simulink library "sim_lib"  (R2023a)
settings: Solver=VariableStepAuto  StartTime=0.0  StopTime=10.0  RelTol=1e-3
undefined symbols (not defined in the file): DiscIntNeverNeededParam, gui, mu, simdb
libraries: $bdroot x12, dspinverses x3, matrix_library x2, simulink x1
settings Model: Creator=David  LastModifiedBy=David
settings OptimizationCC: ReuseModelBlockBuffer=off

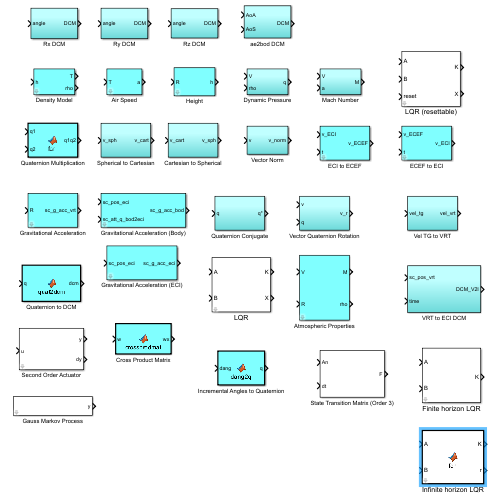
[thumbnail: Simulink's stored preview of the top-level diagram]
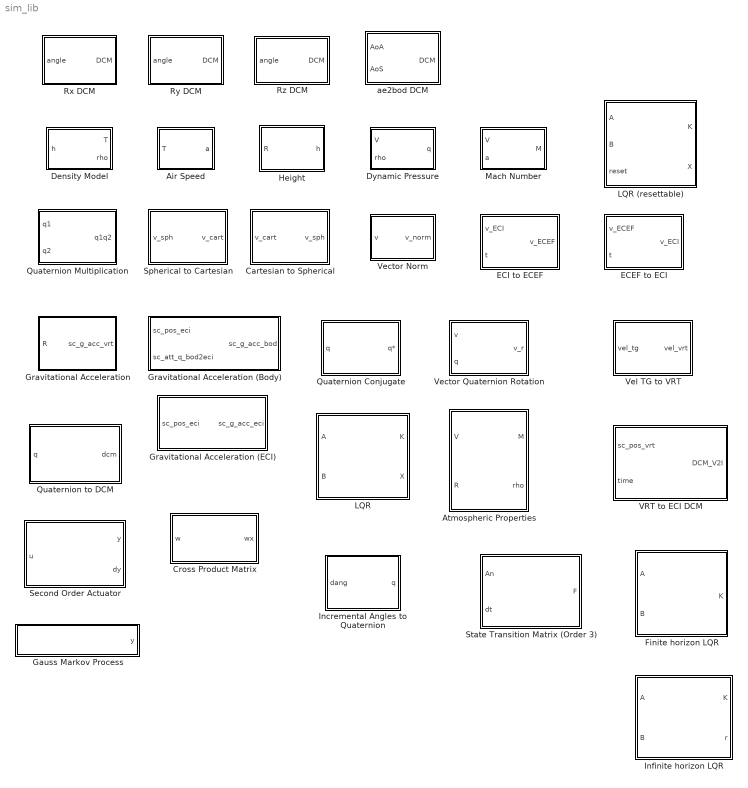
== system sim_lib ==
  Air Speed : Subsystem  mask{Rg=simdb.env.Rg, gamma=simdb.env.gamma}
      mask prompts: Rg "Gas constant"; gamma "Gas constant #2"
  Atmospheric Properties : Subsystem  mask(Atmospheric Properties){Rp=0, Rg=0, gamma=0, h_base=0, T_base=0, rho_base=0}
      mask prompts: Rp "Planet radius [m]:"; Rg "Gas constant (Rg):"; gamma "Gas constant #2 (gamma):"; h_base "Height interpolation breakpoints:"; T_base "Temperature interpolation breakpoints:"; rho_base "Density interpolation breakpoints:"
      mask help: Calculates Mach number and air density at the specified radial position and velocity.
  Cartesian to Spherical : Subsystem
  Cross Product Matrix : MATLAB Function  TreatAsAtomicUnit=on
  Density Model : Subsystem  mask{h_base=simdb.env.h_base, T_base=simdb.env.T_base, rho_base=simdb.env.rho_base}
      mask prompts: h_base "Height breakpoints"; T_base "Temperature interpolation points"; rho_base "Density interpolation points"
  Dynamic Pressure : Subsystem
  ECEF to ECI : Subsystem  mask{omega_cb=0}
      mask prompts: omega_cb "Central body rotation [rad/s]:"
  ECI to ECEF : Subsystem  mask{omega_cb=0}
      mask prompts: omega_cb "Central body rotation [rad/s]:"
  Finite horizon LQR : Subsystem  mask(Linear Quadratic Regulator){Q=gui.Q, R=gui.R, P0=eye(3), T=20, dt=0.05}
      mask prompts: Q "State cost matrix Q:"; R "Input cost matrix R:"; P0 "Initial Ricatti matrix P0:"; T "Time horizon:"; dt "Sample time:"
      mask help: Implementation of the Continuous-Time Finite-Horizon Linear Quadratic Regulator in Simulink (Compatible with Code Generator).
  Gauss Markov Process : Subsystem  mask{var=1, Tc=1, seed=0, dt=1}
      mask prompts: var "Variance:"; Tc "Autocorrelation time [s]:"; dt "Sample time [s]:"
  Gravitational Acceleration : Subsystem  mask{mu=mu}
      mask prompts: mu "Gravitational Parameter [m^3/s^2]:"
  Gravitational Acceleration (Body) : Subsystem  mask{mu=mu}
      mask prompts: mu "Gravitational Parameter [m^3/s^2]:"
  Gravitational Acceleration (ECI) : Subsystem  mask{mu=mu}
      mask prompts: mu "Gravitational Parameter [m^3/s^2]:"
  Height : Subsystem  mask{Rp=simdb.env.Rp}
      mask prompts: Rp "Planet radius"
  Incremental Angles to Quaternion : MATLAB Function  TreatAsAtomicUnit=on
  Infinite horizon LQR : MATLAB Function  TreatAsAtomicUnit=on  mask{Q=simdb.ctl.Q_lat, R=simdb.ctl.R_lat}
      mask prompts: Q "State cost matrix:"; R "Control cost matrix:"
  LQR : Subsystem  mask(Linear Quadratic Regulator){Q=gui.Q, R=gui.R, X0=eye(3)}
      mask prompts: Q "State cost matrix Q:"; R "Input cost matrix R:"; X0 "Initial Ricatti matrix X0 (Identity if unsure):"
      mask help: Implementation of the Continuous-Time Finite-Horizon Linear Quadratic Regulator in Simulink (Compatible with Code Generator).
  LQR (resettable) : Subsystem  mask(Linear Quadratic Regulator){Q=gui.Q, R=gui.R, X0=eye(3)}
      mask prompts: Q "State cost matrix Q:"; R "Input cost matrix R:"; X0 "Initial Ricatti matrix X0 (Identity if unsure):"
      mask help: Implementation of the Continuous-Time Finite-Horizon Linear Quadratic Regulator in Simulink (Compatible with Code Generator).
  Mach Number : Subsystem
  Quaternion Conjugate : Subsystem
  Quaternion Multiplication : MATLAB Function  TreatAsAtomicUnit=on
  Quaternion to DCM : MATLAB Function  TreatAsAtomicUnit=on
  Rx DCM : Subsystem
  Ry DCM : Subsystem
  Rz DCM : Subsystem
  Second Order Actuator : Subsystem  mask{omega=2*pi, chi=0.7, y0=0}
      mask prompts: omega "Natural frequency [rad/s]:"; chi "Damping ratio [-]:"; y0 "Initial conditions:"
  Spherical to Cartesian : Subsystem
  State Transition Matrix (Order 3) : Subsystem
  VRT to ECI DCM : Subsystem
  Vector Norm : Subsystem
  Vector Quaternion Rotation : Subsystem
  Vel TG to VRT : Subsystem
  ae2bod DCM : Subsystem

== system sim_lib/Air Speed ==
  T : Inport
  Product : Product  Inputs=3
  Rg : Constant  Value=Rg
  Sqrt : Sqrt
  gamma : Constant  Value=gamma
  a : Outport
  wires:
  T/1 -> Product/3
  Rg/1 -> Product/1
  gamma/1 -> Product/2
  Product/1 -> Sqrt/1
  Sqrt/1 -> a/1

== system sim_lib/Atmospheric Properties ==
  V : Inport
  R : Inport  Port=2
  Air Speed : $bdroot/Air Speed  Rg=Rg  gamma=gamma
  Atmosphere Model : $bdroot/Density Model  h_base=h_base  T_base=T_base  rho_base=rho_base
  Height : $bdroot/Height  Rp=Rp
  Mach Number : $bdroot/Mach Number  SystemSampleTime=-1  VariantActivationTime=update diagram  Latency=0  AutoFrameSizeCalculation=off
  M : Outport
  rho : Outport  Port=2
  wires:
  Atmosphere Model/2 -> rho/1  "rho"
  Air Speed/1 -> Mach Number/2
  Atmosphere Model/1 -> Air Speed/1
  R/1 -> Height/1
  V/1 -> Mach Number/1
  Height/1 -> Atmosphere Model/1
  Mach Number/1 -> M/1

== system sim_lib/Cartesian to Spherical ==
  v_cart : Inport
  Asin : Trigonometry  Operator=asin
  Atan2 : Trigonometry  Operator=atan2
  Demux : Demux  Outputs=3
  Divide : Product  Inputs=*/
  Mux : Mux  Inputs=3
  Vector Norm : $bdroot/Vector Norm  SystemSampleTime=-1  VariantActivationTime=update diagram  Latency=0  AutoFrameSizeCalculation=off
  v_sph : Outport
  wires:
  v_cart/1 -> Vector Norm/1, Demux/1
  Mux/1 -> v_sph/1
  Vector Norm/1 -> Divide/2, Mux/1  "R"
  Atan2/1 -> Mux/2  "tau"
  Demux/1 -> Atan2/2  "x"
  Demux/2 -> Atan2/1  "y"
  Asin/1 -> Mux/3  "delta"
  Divide/1 -> Asin/1
  Demux/3 -> Divide/1  "z"

== system sim_lib/Density Model ==
  h : Inport
  Density : Interpolation_n-D  NumberOfTableDimensions=1  Table=rho_base  RequireIndexFractionAsBus=on  RemoveProtectionIndex=on  InternalRulePriority=Speed
      settings: InputPortMap=u0
  Temperature : Interpolation_n-D  NumberOfTableDimensions=1  Table=T_base  RequireIndexFractionAsBus=on  RemoveProtectionIndex=on  InternalRulePriority=Speed
      settings: InputPortMap=u0
  h Table : PreLookup  BreakpointsData=h_base  OutputSelection=Index and fraction as bus  BeginIndexSearchUsingPreviousIndexResult=on  ExtrapMethod=Linear  RemoveProtectionInput=on
  T : Outport
  rho : Outport  Port=2
  wires:
  h/1 -> h Table/1
  Density/1 -> rho/1
  Temperature/1 -> T/1
  h Table/1 -> Temperature/1, Density/1

== system sim_lib/Dynamic Pressure ==
  V : Inport
  rho : Inport  Port=2
  Gain : Gain  Gain=0.5
  Product : Product
  Square : Math  Operator=square
  q : Outport
  wires:
  V/1 -> Square/1
  rho/1 -> Product/2
  Square/1 -> Product/1
  Product/1 -> Gain/1
  Gain/1 -> q/1

== system sim_lib/ECEF to ECI ==
  v_ECEF : Inport
  t : Inport  Port=2
  Constant : Constant  Value=omega_cb
  Gain : Gain  Gain=-1
  MatrixMultiply : Product  Multiplication=Matrix(*)
  Product : Product
  Rz DCM : $bdroot/Rz DCM  SystemSampleTime=-1  VariantActivationTime=update diagram  Latency=0  AutoFrameSizeCalculation=off
  v_ECI : Outport
  wires:
  t/1 -> Product/2
  Constant/1 -> Product/1
  Product/1 -> Gain/1
  Rz DCM/1 -> MatrixMultiply/1
  v_ECEF/1 -> MatrixMultiply/2
  MatrixMultiply/1 -> v_ECI/1
  Gain/1 -> Rz DCM/1

== system sim_lib/ECI to ECEF ==
  v_ECI : Inport
  t : Inport  Port=2
  Constant : Constant  Value=omega_cb
  MatrixMultiply : Product  Multiplication=Matrix(*)
  Product : Product
  Rz DCM : $bdroot/Rz DCM  SystemSampleTime=-1  VariantActivationTime=update diagram  Latency=0  AutoFrameSizeCalculation=off
  v_ECEF : Outport
  wires:
  t/1 -> Product/2
  Constant/1 -> Product/1
  Product/1 -> Rz DCM/1
  Rz DCM/1 -> MatrixMultiply/1
  v_ECI/1 -> MatrixMultiply/2
  MatrixMultiply/1 -> v_ECEF/1

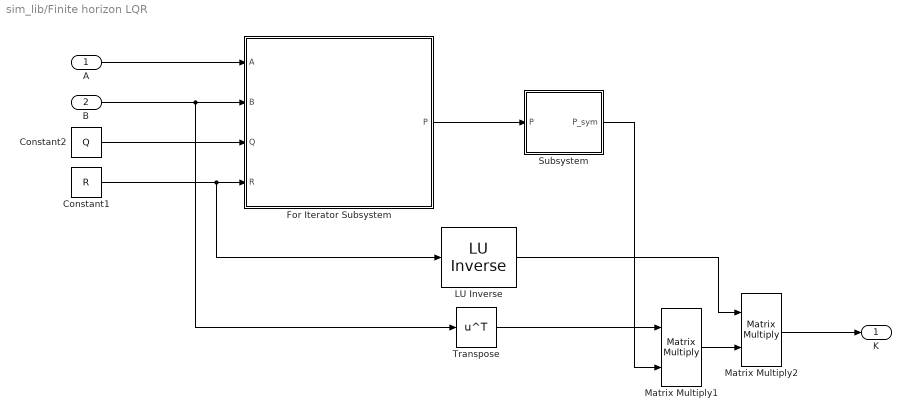
== system sim_lib/Finite horizon LQR ==
  A : Inport
  B : Inport  Port=2
  " LU Inverse" : dspinverses/ LU Inverse
  Constant1 : Constant  Value=R
  Constant2 : Constant  Value=Q
  For Iterator Subsystem : Subsystem  TreatAsAtomicUnit=on
  Matrix Multiply1 : Product  Multiplication=Matrix(*)
  Matrix Multiply2 : Product  Multiplication=Matrix(*)
  Subsystem : Subsystem
  Transpose : Math  Operator=transpose
  K : Outport
  wires:
  Matrix Multiply2/1 -> K/1
  Matrix Multiply1/1 -> Matrix Multiply2/2
  B/1 -> Transpose/1, For Iterator Subsystem/2(B)
  " LU Inverse"/1 -> Matrix Multiply2/1
  Transpose/1 -> Matrix Multiply1/1
  A/1 -> For Iterator Subsystem/1(A)
  Subsystem/1(P_sym) -> Matrix Multiply1/2
  For Iterator Subsystem/1(P) -> Subsystem/1(P)
  Constant2/1 -> For Iterator Subsystem/3(Q)
  Constant1/1 -> " LU Inverse"/1, For Iterator Subsystem/4(R)

== system sim_lib/Gauss Markov Process ==
  (1-dt/Tc) : Gain  Gain=1-dt/Tc
  Delay : Delay  DelayLength=1  SampleTime=dt
  Random Number : RandomNumber  Seed=seed  SampleTime=dt
  Sum : Sum  Inputs=|++
  sqrt(var*(1-exp(-2*dt/Tc))) : Gain  Gain=sqrt(var)*sqrt(1-exp(-2*dt/Tc))
  y : Outport
  wires:
  Random Number/1 -> sqrt(var*(1-exp(-2*dt/Tc)))/1
  Sum/1 -> Delay/1, y/1
  sqrt(var*(1-exp(-2*dt/Tc)))/1 -> Sum/2
  Delay/1 -> (1-dt/Tc)/1
  (1-dt/Tc)/1 -> Sum/1

== system sim_lib/Gravitational Acceleration ==
  R : Inport
  Constant : Constant  Value=mu
  Constant1 : Constant  Value=0
  Constant2 : Constant  Value=0
  Divide : Product  Inputs=*/
  Mux : Mux  Inputs=3
  Square : Math  Operator=square
  sc_g_acc_vrt : Outport
  wires:
  R/1 -> Square/1
  Square/1 -> Divide/2
  Constant/1 -> Divide/1
  Divide/1 -> Mux/3
  Mux/1 -> sc_g_acc_vrt/1
  Constant1/1 -> Mux/1
  Constant2/1 -> Mux/2

== system sim_lib/Gravitational Acceleration (Body) ==
  sc_pos_eci : Inport
  sc_att_q_bod2eci : Inport  Port=2
  Conjugate : $bdroot/Quaternion Conjugate  SystemSampleTime=-1  VariantActivationTime=update diagram  Latency=0  AutoFrameSizeCalculation=off
  Gravitational Acceleration (ECI) : $bdroot/Gravitational Acceleration (ECI)  mu=mu
  Vector Quaternion Rotation : $bdroot/Vector Quaternion Rotation  SystemSampleTime=-1  VariantActivationTime=update diagram  Latency=0  AutoFrameSizeCalculation=off
  sc_g_acc_bod : Outport
  wires:
  sc_att_q_bod2eci/1 -> Conjugate/1
  Vector Quaternion Rotation/1 -> sc_g_acc_bod/1
  Gravitational Acceleration (ECI)/1 -> Vector Quaternion Rotation/1
  Conjugate/1 -> Vector Quaternion Rotation/2  "sc_att_q_eci2bod"
  sc_pos_eci/1 -> Gravitational Acceleration (ECI)/1

== system sim_lib/Gravitational Acceleration (ECI) ==
  sc_pos_eci : Inport
  Constant : Constant  Value=mu
  Constant3 : Constant  Value=3/2
  Divide : Product  Inputs=*/
  Dot Product : DotProduct  OutDataTypeStr=Inherit: Inherit via internal rule
  Gain : Gain  Gain=-1
  Power : Math  Operator=pow
  Product : Product
  sc_g_acc_eci : Outport
  wires:
  Power/1 -> Divide/2
  Constant/1 -> Divide/1
  sc_pos_eci/1 -> Product/1, Dot Product/1, Dot Product/2
  Dot Product/1 -> Power/1
  Constant3/1 -> Power/2
  Divide/1 -> Gain/1
  Gain/1 -> Product/2
  Product/1 -> sc_g_acc_eci/1

== system sim_lib/Height ==
  R : Inport
  Add : Sum  Inputs=-+
  Rp : Constant  Value=Rp
  h : Outport
  wires:
  R/1 -> Add/2
  Rp/1 -> Add/1
  Add/1 -> h/1

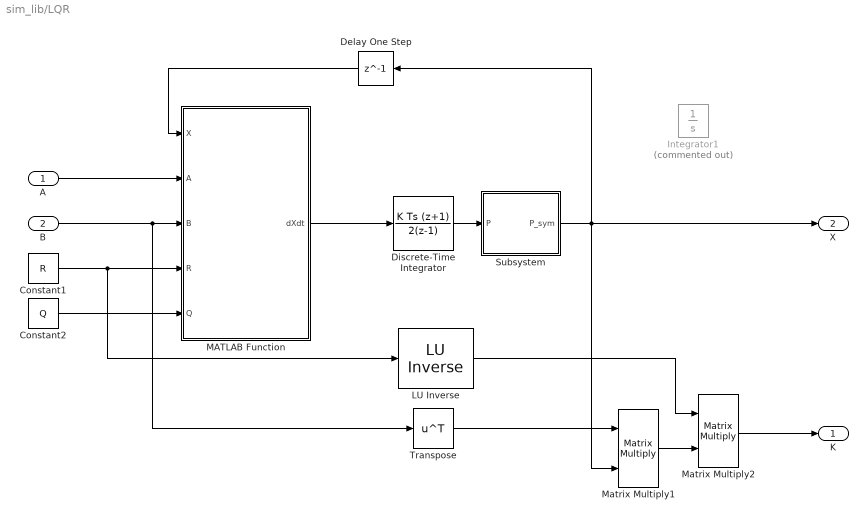
== system sim_lib/LQR ==
  A : Inport
  B : Inport  Port=2
  " LU Inverse" : dspinverses/ LU Inverse
  Constant1 : Constant  Value=R
  Constant2 : Constant  Value=Q
  Delay One Step : Delay  DelayLength=1  InitialCondition=X0
  Discrete-Time Integrator : DiscreteIntegrator  IntegratorMethod=Integration: Trapezoidal  InitialCondition=X0  SampleTime=-1  ICPrevOutput=DiscIntNeverNeededParam  ICPrevScaledInput=DiscIntNeverNeededParam
  Integrator1 : Integrator  Commented=on  InitialConditionSource=external  InitialCondition=[1 1 1 1 1 1 1 1 1 1 1 1 1 1 1 1 1 1 1 1 1 1 1 1 1 1 1 1 1 1 1 1 1 1 1 1]
  MATLAB Function : MATLAB Function  TreatAsAtomicUnit=on
  Matrix Multiply1 : Product  Multiplication=Matrix(*)
  Matrix Multiply2 : Product  Multiplication=Matrix(*)
  Subsystem : Subsystem
  Transpose : Math  Operator=transpose
  K : Outport
  X : Outport  Port=2
  wires:
  Matrix Multiply2/1 -> K/1
  Matrix Multiply1/1 -> Matrix Multiply2/2
  Constant2/1 -> MATLAB Function/5(Q)
  B/1 -> Transpose/1, MATLAB Function/3(B)
  " LU Inverse"/1 -> Matrix Multiply2/1
  Constant1/1 -> " LU Inverse"/1, MATLAB Function/4(R)
  Transpose/1 -> Matrix Multiply1/1
  A/1 -> MATLAB Function/2(A)
  Subsystem/1(P_sym) -> Delay One Step/1, X/1, Matrix Multiply1/2
  Discrete-Time Integrator/1 -> Subsystem/1(P)
  MATLAB Function/1(dXdt) -> Discrete-Time Integrator/1
  Delay One Step/1 -> MATLAB Function/1(X)

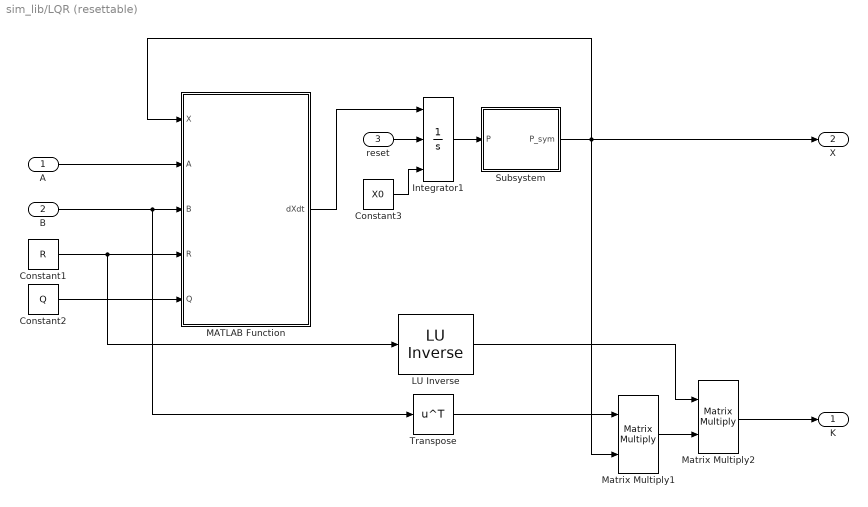
== system sim_lib/LQR (resettable) ==
  A : Inport
  B : Inport  Port=2
  reset : Inport  Port=3
  " LU Inverse" : dspinverses/ LU Inverse
  Constant1 : Constant  Value=R
  Constant2 : Constant  Value=Q
  Constant3 : Constant  Value=X0
  Integrator1 : Integrator  ExternalReset=rising  InitialConditionSource=external  InitialCondition=[1 1 1 1 1 1 1 1 1 1 1 1 1 1 1 1 1 1 1 1 1 1 1 1 1 1 1 1 1 1 1 1 1 1 1 1]
  MATLAB Function : MATLAB Function  TreatAsAtomicUnit=on
  Matrix Multiply1 : Product  Multiplication=Matrix(*)
  Matrix Multiply2 : Product  Multiplication=Matrix(*)
  Subsystem : Subsystem
  Transpose : Math  Operator=transpose
  K : Outport
  X : Outport  Port=2
  wires:
  Matrix Multiply2/1 -> K/1
  Matrix Multiply1/1 -> Matrix Multiply2/2
  Constant2/1 -> MATLAB Function/5(Q)
  B/1 -> Transpose/1, MATLAB Function/3(B)
  Integrator1/1 -> Subsystem/1(P)
  " LU Inverse"/1 -> Matrix Multiply2/1
  Constant1/1 -> " LU Inverse"/1, MATLAB Function/4(R)
  Transpose/1 -> Matrix Multiply1/1
  A/1 -> MATLAB Function/2(A)
  MATLAB Function/1(dXdt) -> Integrator1/1
  Subsystem/1(P_sym) -> MATLAB Function/1(X), X/1, Matrix Multiply1/2
  Constant3/1 -> Integrator1/3
  reset/1 -> Integrator1/2

== system sim_lib/Mach Number ==
  V : Inport
  a : Inport  Port=2
  Divide : Product  Inputs=*/
  M : Outport
  wires:
  V/1 -> Divide/1
  a/1 -> Divide/2
  Divide/1 -> M/1

== system sim_lib/Quaternion Conjugate ==
  q : Inport
  Gain : Gain  Gain=-1
  Mux : Mux  Inputs=2
  Selector : Selector  InputPortWidth=4  IndexOptions=Index vector (dialog)  Indices=[1]  OutputSizes=1
  Selector1 : Selector  InputPortWidth=4  IndexOptions=Index vector (dialog)  Indices=[2 3 4]  OutputSizes=1
  q* : Outport
  wires:
  Mux/1 -> q*/1
  Selector/1 -> Mux/1
  Selector1/1 -> Gain/1
  Gain/1 -> Mux/2
  q/1 -> Selector1/1, Selector/1

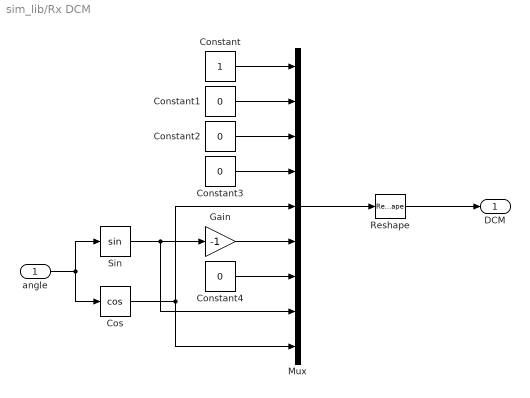
== system sim_lib/Rx DCM ==
  angle : Inport
  Constant : Constant
  Constant{1..4} (4 alike) : Constant  Value=0
  Cos : Trigonometry  Operator=cos
  Gain : Gain  Gain=-1
  Mux : Mux  Inputs=9
  Reshape : Reshape  OutputDimensionality=Customize  OutputDimensions=[3,3]
  Sin : Trigonometry
  DCM : Outport
  wires:
  angle/1 -> Cos/1, Sin/1
  Reshape/1 -> DCM/1
  Mux/1 -> Reshape/1
  Constant/1 -> Mux/1
  Constant1/1 -> Mux/2
  Constant2/1 -> Mux/3
  Constant3/1 -> Mux/4
  Constant4/1 -> Mux/7
  Cos/1 -> Mux/9, Mux/5
  Sin/1 -> Mux/8, Gain/1
  Gain/1 -> Mux/6

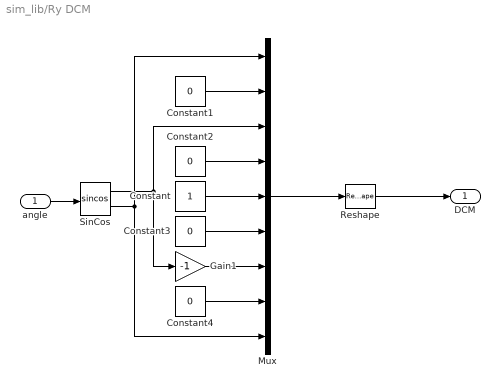
== system sim_lib/Ry DCM ==
  angle : Inport
  Constant : Constant
  Constant{1..4} (4 alike) : Constant  Value=0
  Gain1 : Gain  Gain=-1
  Mux : Mux  Inputs=9
  Reshape : Reshape  OutputDimensionality=Customize  OutputDimensions=[3,3]
  SinCos : Trigonometry  Operator=sincos
  DCM : Outport
  wires:
  angle/1 -> SinCos/1
  Reshape/1 -> DCM/1
  Mux/1 -> Reshape/1
  Constant4/1 -> Mux/8
  Constant3/1 -> Mux/6
  Constant/1 -> Mux/5
  Constant2/1 -> Mux/4
  Constant1/1 -> Mux/2
  SinCos/2 -> Mux/1, Mux/9
  SinCos/1 -> Mux/3, Gain1/1
  Gain1/1 -> Mux/7

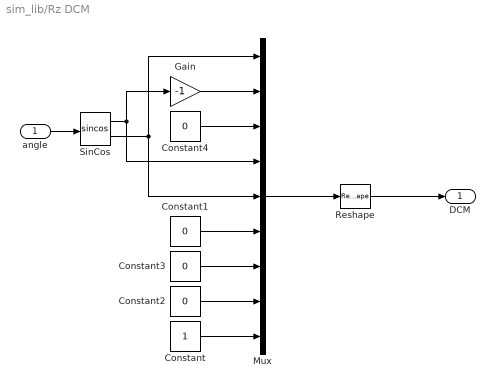
== system sim_lib/Rz DCM ==
  angle : Inport
  Constant : Constant
  Constant{1..4} (4 alike) : Constant  Value=0
  Gain : Gain  Gain=-1
  Mux : Mux  Inputs=9
  Reshape : Reshape  OutputDimensionality=Customize  OutputDimensions=[3,3]
  SinCos : Trigonometry  Operator=sincos
  DCM : Outport
  wires:
  angle/1 -> SinCos/1
  Reshape/1 -> DCM/1
  Mux/1 -> Reshape/1
  Constant/1 -> Mux/9
  Constant3/1 -> Mux/7
  Constant2/1 -> Mux/8
  Constant1/1 -> Mux/6
  Constant4/1 -> Mux/3
  SinCos/2 -> Mux/5, Mux/1
  SinCos/1 -> Mux/4, Gain/1
  Gain/1 -> Mux/2

== system sim_lib/Second Order Actuator ==
  u : Inport
  Add : Sum
  Control Gain : Gain  Gain=[0; omega^2]
  Demux : Demux  Outputs=2
  Integrator : Integrator  InitialCondition=y0
  State Gain : Gain  Gain=[0 1; -omega^2 -2*chi*omega]  Multiplication=Matrix(K*u) (u vector)
  y : Outport
  dy : Outport  Port=2
  wires:
  Integrator/1 -> State Gain/1, Demux/1
  Demux/1 -> y/1
  Demux/2 -> dy/1
  Add/1 -> Integrator/1
  State Gain/1 -> Add/1
  u/1 -> Control Gain/1
  Control Gain/1 -> Add/2

== system sim_lib/Spherical to Cartesian ==
  v_sph : Inport
  Demux : Demux  Outputs=3
  Mux : Mux  Inputs=3
  Product : Product  Inputs=3
  Product1 : Product  Inputs=3
  Product2 : Product
  SinCos : Trigonometry  Operator=sincos
  SinCos1 : Trigonometry  Operator=sincos
  v_cart : Outport
  wires:
  v_sph/1 -> Demux/1
  Mux/1 -> v_cart/1
  Demux/2 -> SinCos/1  "tau"
  Demux/3 -> SinCos1/1  "delta"
  Demux/1 -> Product2/1, Product1/1, Product/1  "R"
  SinCos1/2 -> Product1/2, Product/3
  Product/1 -> Mux/1
  Product1/1 -> Mux/2
  Product2/1 -> Mux/3
  SinCos1/1 -> Product2/2
  SinCos/2 -> Product/2
  SinCos/1 -> Product1/3

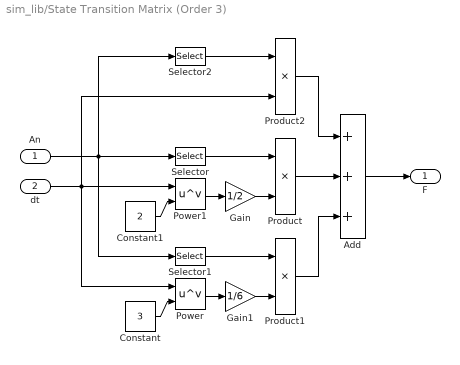
== system sim_lib/State Transition Matrix (Order 3) ==
  An : Inport
  dt : Inport  Port=2
  Add : Sum  Inputs=+++
  Constant : Constant  Value=3
  Constant1 : Constant  Value=2
  Gain : Gain  Gain=1/2
  Gain1 : Gain  Gain=1/6
  Power : Math  Operator=pow
  Power1 : Math  Operator=pow
  Product : Product
  Product1 : Product
  Product2 : Product
  Selector : Selector  NumberOfDimensions=3  InputPortWidth=3  IndexOptions=Select all,Select all,Index vector (dialog)  Indices=[1 3],1,2  OutputSizes=1,1,1
  Selector1 : Selector  NumberOfDimensions=3  InputPortWidth=3  IndexOptions=Select all,Select all,Index vector (dialog)  Indices=[1 3],1,3  OutputSizes=1,1,1
  Selector2 : Selector  NumberOfDimensions=3  InputPortWidth=3  IndexOptions=Select all,Select all,Index vector (dialog)  Indices=[1 3],1,1  OutputSizes=1,1,1
  F : Outport
  wires:
  dt/1 -> Power/1, Power1/1, Product2/2
  Constant/1 -> Power/2
  Constant1/1 -> Power1/2
  Power1/1 -> Gain/1
  Selector/1 -> Product/1
  Selector1/1 -> Product1/1
  Power/1 -> Gain1/1
  Selector2/1 -> Product2/1
  An/1 -> Selector2/1, Selector1/1, Selector/1
  Product/1 -> Add/2
  Product2/1 -> Add/1
  Product1/1 -> Add/3
  Add/1 -> F/1
  Gain/1 -> Product/2
  Gain1/1 -> Product1/2

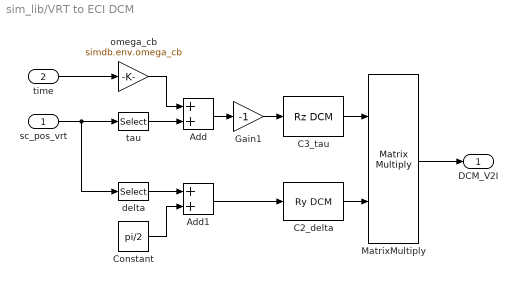
== system sim_lib/VRT to ECI DCM ==
  sc_pos_vrt : Inport
  time : Inport  Port=2
  Add : Sum
  Add1 : Sum
  C2_delta : $bdroot/Ry DCM  SystemSampleTime=-1  VariantActivationTime=update diagram  Latency=0  AutoFrameSizeCalculation=off
  C3_tau : $bdroot/Rz DCM  SystemSampleTime=-1  VariantActivationTime=update diagram  Latency=0  AutoFrameSizeCalculation=off
  Constant : Constant  Value=pi/2
  Gain1 : Gain  Gain=-1
  MatrixMultiply : Product  Multiplication=Matrix(*)
  delta : Selector  InputPortWidth=3  IndexOptions=Index vector (dialog)  Indices=[3]  OutputSizes=1
  omega_cb : Gain  Gain=simdb.env.omega_cb
  tau : Selector  InputPortWidth=3  IndexOptions=Index vector (dialog)  Indices=[2]  OutputSizes=1
  DCM_V2I : Outport
  wires:
  sc_pos_vrt/1 -> delta/1, tau/1
  time/1 -> omega_cb/1
  MatrixMultiply/1 -> DCM_V2I/1
  Add/1 -> Gain1/1
  Gain1/1 -> C3_tau/1
  Add1/1 -> C2_delta/1
  delta/1 -> Add1/1
  Constant/1 -> Add1/2
  C3_tau/1 -> MatrixMultiply/1
  C2_delta/1 -> MatrixMultiply/2
  tau/1 -> Add/2
  omega_cb/1 -> Add/1

== system sim_lib/Vector Norm ==
  v : Inport
  Add : Sum
  Cast To Double : DataTypeConversion  OutDataTypeStr=double  SaturateOnIntegerOverflow=off  RndMeth=Floor
  Compare To Constant : simulink/Logic and Bit Operations/Compare To Constant  relop===  const=0  OutDataTypeStr=uint8
  Dot Product : DotProduct  OutDataTypeStr=Inherit: Inherit via internal rule
  Sqrt : Sqrt
  v_norm : Outport
  wires:
  Sqrt/1 -> Add/2, Compare To Constant/1
  v/1 -> Dot Product/1, Dot Product/2
  Cast To Double/1 -> Add/1
  Compare To Constant/1 -> Cast To Double/1
  Dot Product/1 -> Sqrt/1
  Add/1 -> v_norm/1

== system sim_lib/Vector Quaternion Rotation ==
  v : Inport
  q : Inport  Port=2
  Add : Sum  Inputs=+++
  Cross Product : matrix_library/Cross Product
  Cross Product1 : matrix_library/Cross Product
  Gain : Gain  Gain=2
  Product : Product
  Selector : Selector  InputPortWidth=4  IndexOptions=Index vector (dialog)  Indices=[1]  OutputSizes=1
  Selector1 : Selector  InputPortWidth=4  IndexOptions=Index vector (dialog)  Indices=[2 3 4]  OutputSizes=1
  v_r : Outport
  wires:
  q/1 -> Selector1/1, Selector/1
  Selector1/1 -> Cross Product1/1, Cross Product/1
  v/1 -> Cross Product/2, Add/3
  Cross Product/1 -> Gain/1
  Selector/1 -> Product/1
  Gain/1 -> Cross Product1/2, Product/2
  Product/1 -> Add/1
  Cross Product1/1 -> Add/2
  Add/1 -> v_r/1

== system sim_lib/Vel TG to VRT ==
  vel_tg : Inport
  Demux : Demux  Outputs=3
  Gain : Gain  Gain=-1
  Mux : Mux  Inputs=3
  Product : Product  Inputs=3
  Product1 : Product  Inputs=3
  Product2 : Product
  SinCos : Trigonometry  Operator=sincos
  SinCos1 : Trigonometry  Operator=sincos
  vel_vrt : Outport
  wires:
  vel_tg/1 -> Demux/1
  Mux/1 -> vel_vrt/1
  Demux/2 -> SinCos/1  "gamma"
  Demux/3 -> SinCos1/1  "chi"
  Demux/1 -> Product2/1, Product1/1, Product/1  "V"
  Product/1 -> Mux/1
  Product1/1 -> Mux/2
  Gain/1 -> Mux/3
  Product2/1 -> Gain/1
  SinCos/1 -> Product2/2
  SinCos/2 -> Product/3, Product1/3
  SinCos1/1 -> Product1/2
  SinCos1/2 -> Product/2

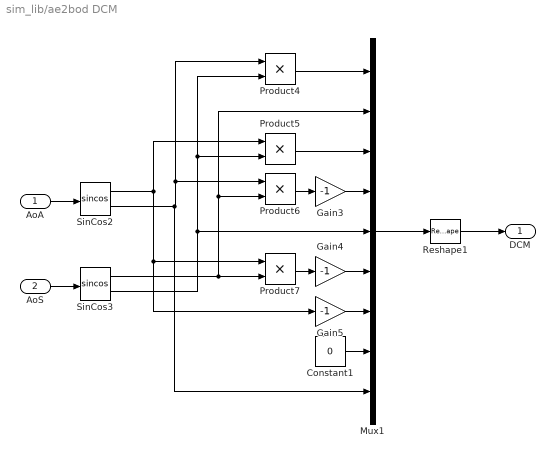
== system sim_lib/ae2bod DCM ==
  AoA : Inport
  AoS : Inport  Port=2
  Constant1 : Constant  Value=0
  Gain3 : Gain  Gain=-1
  Gain4 : Gain  Gain=-1
  Gain5 : Gain  Gain=-1
  Mux1 : Mux  Inputs=9
  Product{4..7} (4 alike) : Product
  Reshape1 : Reshape  OutputDimensionality=Customize  OutputDimensions=[3,3]
  SinCos2 : Trigonometry  Operator=sincos
  SinCos3 : Trigonometry  Operator=sincos
  DCM : Outport
  wires:
  Mux1/1 -> Reshape1/1
  AoS/1 -> SinCos3/1
  AoA/1 -> SinCos2/1
  Reshape1/1 -> DCM/1
  Product4/1 -> Mux1/1
  SinCos2/2 -> Mux1/9, Product6/1, Product4/1
  SinCos3/2 -> Product5/2, Product4/2, Mux1/5
  SinCos3/1 -> Product6/2, Mux1/2, Product7/2
  Product5/1 -> Mux1/3
  SinCos2/1 -> Gain5/1, Product7/1, Product5/1
  Product6/1 -> Gain3/1
  Gain3/1 -> Mux1/4
  Gain4/1 -> Mux1/6
  Product7/1 -> Gain4/1
  Gain5/1 -> Mux1/7
  Constant1/1 -> Mux1/8

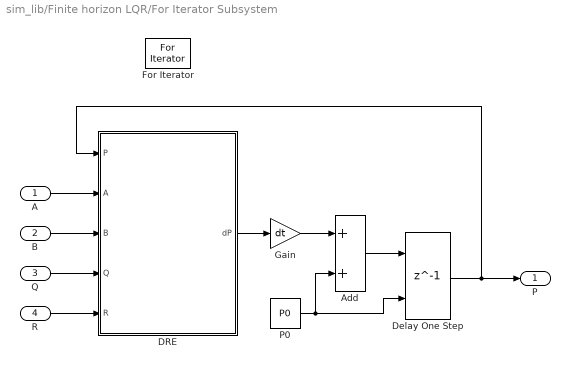
== system sim_lib/Finite horizon LQR/For Iterator Subsystem ==
  A : Inport
  B : Inport  Port=2
  Q : Inport  Port=3
  R : Inport  Port=4
  Add : Sum
  DRE : Subsystem
  Delay One Step : Delay  DelayLength=1  InitialConditionSource=Input port
      settings: InputPortMap=u0,p4
  For Iterator : ForIterator  ResetStates=reset  IterationLimit=T/dt  ShowIterationPort=off
  Gain : Gain  Gain=dt
  P0 : Constant  Value=P0
  P : Outport
  wires:
  DRE/1(dP) -> Gain/1
  A/1 -> DRE/2(A)
  B/1 -> DRE/3(B)
  Q/1 -> DRE/4(Q)
  R/1 -> DRE/5(R)
  Delay One Step/1 -> P/1, DRE/1(P)
  P0/1 -> Add/2, Delay One Step/2
  Add/1 -> Delay One Step/1
  Gain/1 -> Add/1

== system sim_lib/Finite horizon LQR/Subsystem ==
  P : Inport
  Add : Sum
  Gain : Gain  Gain=0.5
  Transpose : Math  Operator=transpose
  P_sym : Outport
  wires:
  P/1 -> Transpose/1, Add/2
  Transpose/1 -> Add/1
  Add/1 -> Gain/1
  Gain/1 -> P_sym/1

== system sim_lib/LQR/Subsystem ==
  P : Inport
  Add : Sum
  Gain : Gain  Gain=0.5
  Transpose : Math  Operator=transpose
  P_sym : Outport
  wires:
  P/1 -> Transpose/1, Add/2
  Transpose/1 -> Add/1
  Add/1 -> Gain/1
  Gain/1 -> P_sym/1

== system sim_lib/LQR (resettable)/Subsystem ==
  P : Inport
  Add : Sum
  Gain : Gain  Gain=0.5
  Transpose : Math  Operator=transpose
  P_sym : Outport
  wires:
  P/1 -> Transpose/1, Add/2
  Transpose/1 -> Add/1
  Add/1 -> Gain/1
  Gain/1 -> P_sym/1

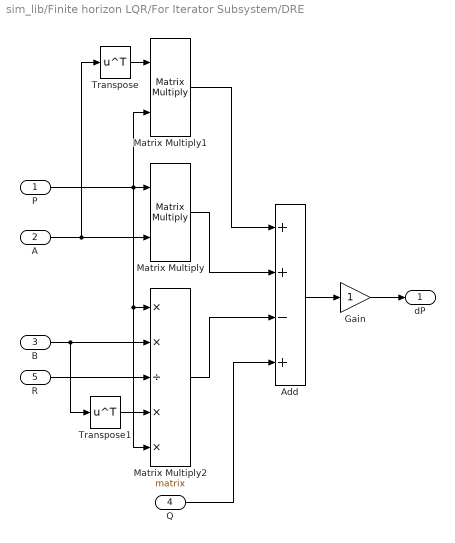
== system sim_lib/Finite horizon LQR/For Iterator Subsystem/DRE ==
  P : Inport
  A : Inport  Port=2
  B : Inport  Port=3
  Q : Inport  Port=4
  R : Inport  Port=5
  Add : Sum  Inputs=++-+
  Gain : Gain
  Matrix Multiply : Product  Multiplication=Matrix(*)
  Matrix Multiply1 : Product  Multiplication=Matrix(*)
  Matrix Multiply2 : Product  Inputs=**/**  Multiplication=Matrix(*)
  Transpose : Math  Operator=transpose
  Transpose1 : Math  Operator=transpose
  dP : Outport
  wires:
  A/1 -> Transpose/1, Matrix Multiply/2
  P/1 -> Matrix Multiply1/2, Matrix Multiply2/5, Matrix Multiply2/1, Matrix Multiply/1
  Transpose/1 -> Matrix Multiply1/1
  B/1 -> Matrix Multiply2/2, Transpose1/1
  Transpose1/1 -> Matrix Multiply2/4
  R/1 -> Matrix Multiply2/3
  Matrix Multiply1/1 -> Add/1
  Matrix Multiply/1 -> Add/2
  Matrix Multiply2/1 -> Add/3
  Q/1 -> Add/4
  Add/1 -> Gain/1
  Gain/1 -> dP/1

== matlab function sim_lib/Quaternion to DCM ==
  data: q input; dcm output
function dcm = quat2dcm(q)
    dcm = zeros(3,3);

    qww = q(1)^2; qwx = q(1)*q(2); qwy = q(1)*q(3); qwz = q(1)*q(4);
    qxx = q(2)^2; qxy = q(2)*q(3); qxz = q(2)*q(4);
    qyy = q(3)^2; qyz = q(3)*q(4);
    qzz = q(4)^2;

    dcm = [qww+qxx-qyy-qzz    2*(qxy - qwz)    2*(qwy + qxz);
             2*(qxy + qwz)  qww-qxx+qyy-qzz    2*(qyz - qwx);
             2*(qxz - qwy)    2*(qwx + qyz)  qww-qxx-qyy+qzz];
end

== matlab function sim_lib/Quaternion Multiplication ==
  data: q1 input; q1q2 output; q2 input
function q1q2 = fcn(q1, q2)

q1q2 = zeros(4,1);
q1q2 = [q1(1)*q2(1) - q1(2)*q2(2) - q1(3)*q2(3) - q1(4)*q2(4);
        q1(1)*q2(2) + q1(2)*q2(1) + q1(3)*q2(4) - q1(4)*q2(3);
        q1(1)*q2(3) - q1(2)*q2(4) + q1(3)*q2(1) + q1(4)*q2(2);
        q1(1)*q2(4) + q1(2)*q2(3) - q1(3)*q2(2) + q1(4)*q2(1)];

== matlab function sim_lib/Cross Product Matrix ==
  data: w input; wx output
function wx = crossprodmat(w)
    wx = [0 -w(3) w(2); w(3) 0 -w(1); -w(2) w(1) 0];
end

== matlab function sim_lib/Incremental Angles to Quaternion ==
  data: dang input; q output
function q = dang2q(dang)
    q = zeros(4,1);
    U = norm(dang);
    u = dang / (U + (U==0));
    q = [cos(U/2); u*sin(U/2)];
end

== matlab function sim_lib/LQR/MATLAB Function ==
  data: dXdt output; X input; A input; B input; R input; Q input
function dXdt  = mRiccati(X, A, B,R,Q)

dXdt = zeros(size(A));
dXdt = (A.'*X + X*A - (X*B)*inv(R)*(B.'*X) + Q); %Determine derivative

== matlab function sim_lib/LQR (resettable)/MATLAB Function ==
  data: dXdt output; X input; A input; B input; R input; Q input
function dXdt  = mRiccati(X, A, B,R,Q)

dXdt = zeros(size(A));
dXdt = (A.'*X + X*A - (X*B)*inv(R)*(B.'*X) + Q); %Determine derivative

== matlab function sim_lib/Infinite horizon LQR ==
  data: A input; K output; B input; Q parameter; R parameter; r output
function [K, r] = fcn(A, B, Q, R)
    rows = size(B,2);
    cols = size(A,1);
    K = zeros(rows,cols);

    Cb = ctrl(A,B);
    r = rank(Cb);

    if r == cols
        K = lqr(A,B,Q,R);
    end
end
